simulink model "QRLsimbranch"  (R2013b)
settings: Solver=ode3  StartTime=0.0  StopTime=Tsim_end  FixedStep=Tsim_s  RelTol=1e-3
values from neighbouring files (symbols this model uses):
  b = 0.1    [QRLrunfile.m]    (also in hat.m = vec(2))
  b1d = [1; 0; 0]    [QRLrunfile.m]
  ctauf = 8.004e-3    (= 0.008004)    [QRLrunfile.m]
  d = 0.1    [QRLrunfile.m]
  dq0 = [0;0;0]    [QRLrunfile.m]
  dxL0 = 0    [QRLrunfile.m]
  dyL0 = 0    [QRLrunfile.m]
  dzL0 = 0    [QRLrunfile.m]
  e3 = [0;0;1]    [QRLrunfile.m]
  fsat = 4*1.96*[1 -1]    [QRLrunfile.m]
  g = 9.81    [LQRrunfile.m]    (also in QRLrunfile.m)
  I = diag([Ixx Iyy Izz])    [QRLrunfile.m]
  Ir = 0.5    [QRLrunfile.m]
  Ixx = 0.0820    (= 0.082)    [LQRrunfile.m]    (also in QRLrunfile.m = 0.00223)
  Iyy = 0.0845    [LQRrunfile.m]    (also in QRLrunfile.m = 0.00299)
  Izz = 0.1377    [LQRrunfile.m]    (also in QRLrunfile.m = 0.0048)
  K = lqr(LQRA,LQRB,LQRQ,LQRR)    [LQRrunfile.m]
  kdx = 2.75    [QRLrunfile.m]
  komega = 0.1    [QRLQRATT-18-Apr-2017.mat]    (also in QRLrunfile.m = 2; savename.mat)
  kOmega = 0.1    [QRLrunfile.m]
  kpx = 6    [QRLrunfile.m]
  kq = 4    [QRLQRATT-18-Apr-2017.mat]    (also in QRLrunfile.m = 3.9; savename.mat)
  kR = 8.81    [QRLQRATT-18-Apr-2017.mat]    (also in QRLrunfile.m = 0.9; savename.mat)
  L = 0.7    [QRLrunfile.m]
  l = 0.126    [QRLrunfile.m]
  LQRA = [zeros(8) eye(8) ... (first row only)    [LQRrunfile.m]
  LQRB = [zeros(10,4) ... (first row only)    [LQRrunfile.m]
  LQRC = eye(16)    [LQRrunfile.m]
  mL = 0.1    [LQRrunfile.m]    (also in QRLrunfile.m)
  mode = 4    [QRLrunfile.m]
  mQ = 4.34    [LQRrunfile.m]    (also in QRLrunfile.m = 0.4)
  Msat = 2*l*1.96*[1 -1]    [QRLrunfile.m]
  phiL0 = deg2rad(0)    [QRLrunfile.m]
  pQ0 = 0    [QRLrunfile.m]
  psiL0 = 0    [QRLrunfile.m]
  q0 = [0 0 -1]    [QRLQRATT-18-Apr-2017.mat]    (also in QRLrunfile.m = Rzyx*e3*qmode; savename.mat)
  qd = [0; 0; qmode]    [QRLrunfile.m]
  qmode = -1    [QRLrunfile.m]
  qQ0 = 0    [QRLrunfile.m]
  R0 = [1  0  0; 0  0.5  -0.866025403784; 0  0.866025403784  0.5]    [QRLQRATT-18-Apr-2017.mat]    (also in QRLrunfile.m = Rzyx; savename.mat)
  Rd = eye(3)    [QRLrunfile.m]
  rQ0 = 0    [QRLrunfile.m]
  stepamp = 0.25    [QRLrunfile.m]
  stept = 1    [QRLrunfile.m]
  thetaL0 = deg2rad(0)    [QRLrunfile.m]
  xL0 = q0(1)*L    [QRLrunfile.m]
  yL0 = q0(2)*L    [QRLrunfile.m]
  zL0 = L+q0(3)*L    [QRLrunfile.m]
undefined symbols (not defined in the file or in its folder): lqr0, sigbuilder_block, T0
libraries: simulink_extras x8, CF3 x7, vrlib x5, simulink x5, dspmathops x3, aerolibtransform2 x2, CommandFilter x1
(part 2 of 2)

== system QRLsimbranch/Trajectory/Path/Sines/Sine diagonal ==
  Add : Sum
  Add1 : Sum
  Add2 : Sum
  Gain : Gain
  Gain1 : Gain
  Gain2 : Gain
  Mux1 : Mux  Inputs=3
  Product : Product
  Product2 : Product
  Product6 : Product
  Scope3 : Scope  NumInputPorts=3
      settings: YMin=-5~-5~-5  YMax=5~5~5  SaveName=ScopeData24
  Signal Builder : Subsystem  Tag=STV Subsys  LoadFcn=sigbuilder_block('load');  StartFcn=sigbuilder_block('start');  StopFcn=sigbuilder_block('stop');  ClipboardFcn=sigbuilder_block('clipboard');  mask(Sigbuilder block){}
      mask help: Simulink:masks:SigbuilderBlock_MD
      mask init:
      | if ~strcmp(get_param(bdroot(gcbh),'SimulationStatus'),'stopped') tuvar = sigbuilder_block('maskInit'); end
      settings: CopyFcn=sigbuilder_block('copy');  DeleteFcn=sigbuilder_block('delete');  ModelCloseFcn=sigbuilder_block('modelClose');  PreSaveFcn=sigbuilder_block('preSave');  PauseFcn=sigbuilder_block('pause');  ContinueFcn=sigbuilder_block('continue');  NameChangeFcn=sigbuilder_block('namechange');  OpenFcn=sigbuilder_block('open',[0 222 1024.5 489 ]);  CloseFcn=sigbuilder_block('close');
      mask Display: plot(0, 0, 100, 100,[2, 2, 32, 32, 2], [68, 8, 8, 68, 68],[32, 2], [38, 38], [32, 19, 2],[53, 60, 44], [32, 17, 17, 2],[16, 16, 31, 31]);txt = getActiveGroup(gcbh);text(2, 100, txt,'verticalAlignment', 'top');
  Sine Wave7 : Sin  Bias=1  Frequency=2*pi/20  Phase=pi  SampleTime=0
  Sine Wave8 : Sin  Amplitude=0.25  Bias=0.25  Frequency=2*pi/3  SampleTime=0
  Sine Wave9 : Sin  Amplitude=0.25  Bias=0.25  Frequency=2*pi/3  SampleTime=0
  Out1 : Outport
  wires:
  Sine Wave7/1 -> Product/1, Scope3/1
  Add2/1 -> Gain/1
  Mux1/1 -> Out1/1
  Signal Builder/3(Signal 3) -> Product2/2
  Signal Builder/2(Signal 2) -> Add/2
  Product6/1 -> Add2/1
  Add/1 -> Gain2/1
  Signal Builder/1(Signal 1) -> Product/2
  Product/1 -> Add/1
  Gain/1 -> Mux1/3
  Sine Wave9/1 -> Scope3/3, Product6/1
  Add1/1 -> Gain1/1
  Gain1/1 -> Mux1/2
  Signal Builder/5(Signal 5) -> Product6/2
  Product2/1 -> Add1/1
  Sine Wave8/1 -> Product2/1, Scope3/2
  Gain2/1 -> Mux1/1

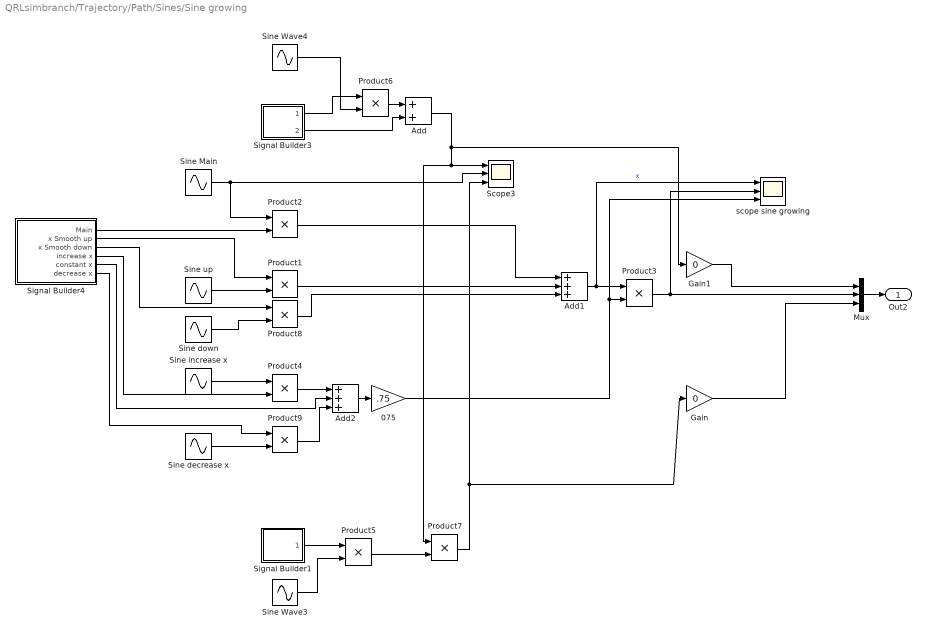
== system QRLsimbranch/Trajectory/Path/Sines/Sine growing ==
  075 : Gain  Gain=.75
  Add : Sum
  Add1 : Sum  Inputs=+++
  Add2 : Sum  Inputs=+++
  Gain : Gain  Gain=0
  Gain1 : Gain  Gain=0
  Mux : Mux  Inputs=3
  Product{1..9} (9 alike) : Product
  Scope3 : Scope  NumInputPorts=3
      settings: YMin=0~-1~0  YMax=0.9~1~0.45  SaveName=ScopeData54
  Signal Builder1 : Subsystem  Tag=STV Subsys  LoadFcn=sigbuilder_block('load');  StartFcn=sigbuilder_block('start');  StopFcn=sigbuilder_block('stop');  ClipboardFcn=sigbuilder_block('clipboard');  mask(Sigbuilder block){}
      mask help: Simulink:masks:SigbuilderBlock_MD
      mask init:
      | if ~strcmp(get_param(bdroot(gcbh),'SimulationStatus'),'stopped') tuvar = sigbuilder_block('maskInit'); end
      settings: CopyFcn=sigbuilder_block('copy');  DeleteFcn=sigbuilder_block('delete');  ModelCloseFcn=sigbuilder_block('modelClose');  PreSaveFcn=sigbuilder_block('preSave');  PauseFcn=sigbuilder_block('pause');  ContinueFcn=sigbuilder_block('continue');  NameChangeFcn=sigbuilder_block('namechange');  OpenFcn=sigbuilder_block('open',[6 28.5 1012.5 484.5 ]);  CloseFcn=sigbuilder_block('close');
      mask Display: plot(0, 0, 100, 100,[2, 2, 32, 32, 2], [68, 8, 8, 68, 68],[32, 2], [38, 38], [32, 19, 2],[53, 60, 44], [32, 17, 17, 2],[16, 16, 31, 31]);txt = getActiveGroup(gcbh);text(2, 100, txt,'verticalAlignment', 'top');
  Signal Builder3 : Subsystem  Tag=STV Subsys  LoadFcn=sigbuilder_block('load');  StartFcn=sigbuilder_block('start');  StopFcn=sigbuilder_block('stop');  ClipboardFcn=sigbuilder_block('clipboard');  mask(Sigbuilder block){}
      mask help: Simulink:masks:SigbuilderBlock_MD
      mask init:
      | if ~strcmp(get_param(bdroot(gcbh),'SimulationStatus'),'stopped') tuvar = sigbuilder_block('maskInit'); end
      settings: CopyFcn=sigbuilder_block('copy');  DeleteFcn=sigbuilder_block('delete');  ModelCloseFcn=sigbuilder_block('modelClose');  PreSaveFcn=sigbuilder_block('preSave');  PauseFcn=sigbuilder_block('pause');  ContinueFcn=sigbuilder_block('continue');  NameChangeFcn=sigbuilder_block('namechange');  OpenFcn=sigbuilder_block('open',[6 28.5 1012.5 484.5 ]);  CloseFcn=sigbuilder_block('close');
      mask Display: plot(0, 0, 100, 100,[2, 2, 32, 32, 2], [68, 8, 8, 68, 68],[32, 2], [38, 38], [32, 19, 2],[53, 60, 44], [32, 17, 17, 2],[16, 16, 31, 31]);txt = getActiveGroup(gcbh);text(2, 100, txt,'verticalAlignment', 'top');
  Signal Builder4 : Subsystem  Tag=STV Subsys  LoadFcn=sigbuilder_block('load');  StartFcn=sigbuilder_block('start');  StopFcn=sigbuilder_block('stop');  ClipboardFcn=sigbuilder_block('clipboard');  mask(Sigbuilder block){}
      mask help: Simulink:masks:SigbuilderBlock_MD
      mask init:
      | if ~strcmp(get_param(bdroot(gcbh),'SimulationStatus'),'stopped') tuvar = sigbuilder_block('maskInit'); end
      settings: CopyFcn=sigbuilder_block('copy');  DeleteFcn=sigbuilder_block('delete');  ModelCloseFcn=sigbuilder_block('modelClose');  PreSaveFcn=sigbuilder_block('preSave');  PauseFcn=sigbuilder_block('pause');  ContinueFcn=sigbuilder_block('continue');  NameChangeFcn=sigbuilder_block('namechange');  OpenFcn=sigbuilder_block('open',[518.25 228 500.25 477 ]);  CloseFcn=sigbuilder_block('close');
      mask Display: plot(0, 0, 100, 100,[2, 2, 32, 32, 2], [68, 8, 8, 68, 68],[32, 2], [38, 38], [32, 19, 2],[53, 60, 44], [32, 17, 17, 2],[16, 16, 31, 31]);txt = getActiveGroup(gcbh);text(2, 100, txt,'verticalAlignment', 'top');
  Sine Main : Sin  Frequency=2*pi/3  SampleTime=0
  Sine Wave3 : Sin  Amplitude=0.5/2  Bias=0.5/2  Frequency=2*pi/1.5  Phase=1.5*pi  SampleTime=0
  Sine Wave4 : Sin  Amplitude=0.5  Bias=0.5  Frequency=2*pi/40  Phase=1.5*pi  SampleTime=0
  Sine decrease x : Sin  Amplitude=.5  Bias=.5  Frequency=2*pi/20  Phase=1*pi  SampleTime=0
  Sine down : Sin  Amplitude=.5  Bias=.5  Frequency=2*pi/3  Phase=0*pi  SampleTime=0
  Sine increase x : Sin  Amplitude=.5  Bias=.5  Frequency=2*pi/20  Phase=1.5*pi  SampleTime=0
  Sine up : Sin  Amplitude=.5  Bias=.5  Frequency=2*pi/1.5  Phase=1.5*pi  SampleTime=0
  scope sine growing : Scope  NumInputPorts=3
      settings: YMin=-5~-5~-5  YMax=5~5~5  SaveName=ScopeData55
  Out2 : Outport
  wires:
  Add1/1 -> scope sine growing/1, Product3/1  "x"
  Product2/1 -> Add1/1
  Sine Main/1 -> Scope3/2, Product2/1
  Product1/1 -> Add1/2
  Product3/1 -> scope sine growing/2, Mux/2
  Mux/1 -> Out2/1
  Add2/1 -> 075/1
  Signal Builder1/1(Signal 3) -> Product5/1
  Sine Wave3/1 -> Product5/2
  Signal Builder3/1(Signal 3) -> Product6/1
  Sine Wave4/1 -> Product6/2
  Product6/1 -> Add/1
  Signal Builder3/2(Signal 1) -> Add/2
  Add/1 -> Product7/1, Scope3/1, Gain1/1
  Gain1/1 -> Mux/1
  Product7/1 -> Scope3/3, Gain/1
  Gain/1 -> Mux/3
  Product5/1 -> Product7/2
  Signal Builder4/1(Main) -> Product2/2
  Signal Builder4/2(x Smooth up) -> Product1/1
  Sine up/1 -> Product1/2
  Product8/1 -> Add1/3
  Signal Builder4/3(x Smooth down) -> Product8/1
  Sine down/1 -> Product8/2
  Product4/1 -> Add2/1
  Sine increase x/1 -> Product4/1
  Signal Builder4/4(increase x) -> Product4/2
  Sine decrease x/1 -> Product9/2
  075/1 -> scope sine growing/3, Product3/2
  Signal Builder4/6(decrease x) -> Product9/1
  Signal Builder4/5(constant x) -> Add2/2
  Product9/1 -> Add2/3

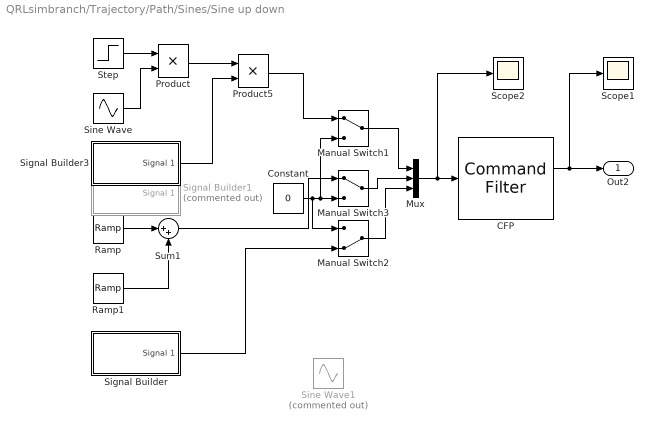
== system QRLsimbranch/Trajectory/Path/Sines/Sine up down ==
  CFP : CF3/Command Filter  Integrator1_init=0  omega_n1=omega_n1_CFP  omega_n2=omega_n2_CFP  zeta=zeta_xL
  Constant : Constant  Value=0
  Manual Switch1 : ManualSwitch
  Manual Switch2 : ManualSwitch  CurrentSetting=0
  Manual Switch3 : ManualSwitch
  Mux : Mux  Inputs=3
  Product : Product
  Product5 : Product
  Ramp : simulink/Sources/Ramp  slope=1/2  start=0  X0=0
  Ramp1 : simulink/Sources/Ramp  slope=-1/2  start=14  X0=0
  Scope1 : Scope
      settings: SaveName=ScopeData8
  Scope2 : Scope
      settings: SaveName=ScopeData50
  Signal Builder : Subsystem  Tag=STV Subsys  LoadFcn=sigbuilder_block('load');  StartFcn=sigbuilder_block('start');  StopFcn=sigbuilder_block('stop');  ClipboardFcn=sigbuilder_block('clipboard');  mask(Sigbuilder block){}
      mask help: Simulink:masks:SigbuilderBlock_MD
      mask init:
      | if ~strcmp(get_param(bdroot(gcbh),'SimulationStatus'),'stopped') tuvar = sigbuilder_block('maskInit'); end
      settings: CopyFcn=sigbuilder_block('copy');  DeleteFcn=sigbuilder_block('delete');  ModelCloseFcn=sigbuilder_block('modelClose');  PreSaveFcn=sigbuilder_block('preSave');  PauseFcn=sigbuilder_block('pause');  ContinueFcn=sigbuilder_block('continue');  NameChangeFcn=sigbuilder_block('namechange');  OpenFcn=sigbuilder_block('open',[611.25 186.75 750 399.75 ]);  CloseFcn=sigbuilder_block('close');
      mask Display: plot(0, 0, 100, 100,[2, 2, 32, 32, 2], [68, 8, 8, 68, 68],[32, 2], [38, 38], [32, 19, 2],[53, 60, 44], [32, 17, 17, 2],[16, 16, 31, 31]);txt = getActiveGroup(gcbh);text(2, 100, txt,'verticalAlignment', 'top');
  Signal Builder1 : Subsystem  Tag=STV Subsys  Commented=on  LoadFcn=sigbuilder_block('load');  StartFcn=sigbuilder_block('start');  StopFcn=sigbuilder_block('stop');  ClipboardFcn=sigbuilder_block('clipboard');  mask(Sigbuilder block){}
      mask help: Simulink:masks:SigbuilderBlock_MD
      mask init:
      | if ~strcmp(get_param(bdroot(gcbh),'SimulationStatus'),'stopped') tuvar = sigbuilder_block('maskInit'); end
      settings: CopyFcn=sigbuilder_block('copy');  DeleteFcn=sigbuilder_block('delete');  ModelCloseFcn=sigbuilder_block('modelClose');  PreSaveFcn=sigbuilder_block('preSave');  PauseFcn=sigbuilder_block('pause');  ContinueFcn=sigbuilder_block('continue');  NameChangeFcn=sigbuilder_block('namechange');  OpenFcn=sigbuilder_block('open',[6 213.75 948 395.25 ]);  CloseFcn=sigbuilder_block('close');
      mask Display: plot(0, 0, 100, 100,[2, 2, 32, 32, 2], [68, 8, 8, 68, 68],[32, 2], [38, 38], [32, 19, 2],[53, 60, 44], [32, 17, 17, 2],[16, 16, 31, 31]);txt = getActiveGroup(gcbh);text(2, 100, txt,'verticalAlignment', 'top');
  Signal Builder3 : Subsystem  Tag=STV Subsys  LoadFcn=sigbuilder_block('load');  StartFcn=sigbuilder_block('start');  StopFcn=sigbuilder_block('stop');  ClipboardFcn=sigbuilder_block('clipboard');  mask(Sigbuilder block){}
      mask help: Simulink:masks:SigbuilderBlock_MD
      mask init:
      | if ~strcmp(get_param(bdroot(gcbh),'SimulationStatus'),'stopped') tuvar = sigbuilder_block('maskInit'); end
      settings: CopyFcn=sigbuilder_block('copy');  DeleteFcn=sigbuilder_block('delete');  ModelCloseFcn=sigbuilder_block('modelClose');  PreSaveFcn=sigbuilder_block('preSave');  PauseFcn=sigbuilder_block('pause');  ContinueFcn=sigbuilder_block('continue');  NameChangeFcn=sigbuilder_block('namechange');  OpenFcn=sigbuilder_block('open',[6 213.75 948 395.25 ]);  CloseFcn=sigbuilder_block('close');
      mask Display: plot(0, 0, 100, 100,[2, 2, 32, 32, 2], [68, 8, 8, 68, 68],[32, 2], [38, 38], [32, 19, 2],[53, 60, 44], [32, 17, 17, 2],[16, 16, 31, 31]);txt = getActiveGroup(gcbh);text(2, 100, txt,'verticalAlignment', 'top');
  Sine Wave : Sin  Frequency=2*pi/2.5  SampleTime=0
  Sine Wave1 : Sin  Commented=on  Frequency=2*pi/2.5*2  Phase=pi  SampleTime=0
  Step : Step  Time=0  After=.5  SampleTime=0
  Sum1 : Sum  Inputs=|++
  Out2 : Outport
  wires:
  Mux/1 -> Scope2/1, CFP/1
  Constant/1 -> Manual Switch3/2, Manual Switch1/2, Manual Switch2/1
  Manual Switch1/1 -> Mux/1
  Manual Switch2/1 -> Mux/3
  Ramp/1 -> Sum1/1
  Manual Switch3/1 -> Mux/2
  Step/1 -> Product/1
  Sine Wave/1 -> Product/2
  Product/1 -> Product5/1
  Product5/1 -> Manual Switch1/1
  Ramp1/1 -> Sum1/2
  Sum1/1 -> Manual Switch3/1
  CFP/2 -> Scope1/1, Out2/1
  Signal Builder/1(Signal 1) -> Manual Switch2/2
  Signal Builder3/1(Signal 1) -> Product5/2

== system QRLsimbranch/Trajectory/Path/Square/Signal Builder3 ==
  Demux : Demux  Tag=STV Demux  Outputs=2
  FromWs : FromWorkspace  Tag=STV FromWs  VariableName=tuvar  SampleTime=0
      SigBuilderData=|
      | common.afterFinalStr = 'Extrapolate'
      | common.sampleTime = 0
      | dataSet.timeRange = [0 20]
      | dataSet.name = 'Group 1'
      | sbobj.Groups.Name = 'Group 1'
      | sbobj.Groups.Signals(1).Name = 'Signal 1'
      | sbobj.Groups.Signals(1).XData = [0 1 5 9 13 20]
      | sbobj.Groups.Signals(1).YData = [0 0 1 1 0 0]
      | sbobj.Groups.Signals(2).Name = 'Signal 2'
      | sbobj.Groups.Signals(2).XData = [0 5 9 13 17 20]
      | sbobj.Groups.Signals(2).YData = [0 0 1 1 0 0]
      | sbobj.Groups.TimeRange = [0 20]
  Signal 1 : Outport  Tag=STV Outport
  Signal 2 : Outport  Tag=STV Outport  Port=2
  wires:
  Demux/1 -> Signal 1/1
  FromWs/1 -> Demux/1
  Demux/2 -> Signal 2/1

== system QRLsimbranch/Trajectory/Step/step3dir/Signal Builder ==
  Demux : Demux  Tag=STV Demux  Outputs=6
  FromWs : FromWorkspace  Tag=STV FromWs  VariableName=tuvar  SampleTime=0
      SigBuilderData=|
      | common.afterFinalStr = 'Extrapolate'
      | common.sampleTime = 0
      | dataSet.timeRange = [0 15]
      | dataSet.name = 'Group 1'
      | sbobj.Groups.Name = 'Group 1'
      | sbobj.Groups.Signals(1).Name = 'Signal 1'
      | sbobj.Groups.Signals(1).XData = [0 1 1 4 4 15]
      | sbobj.Groups.Signals(1).YData = [0 0 1 1 0 0]
      | sbobj.Groups.Signals(2).Name = 'Signal 2'
      | sbobj.Groups.Signals(2).XData = [0 4 4 15]
      | sbobj.Groups.Signals(2).YData = [0 0 1 1]
      | sbobj.Groups.Signals(3).Name = 'Signal 3'
      | sbobj.Groups.Signals(3).XData = [0 4.5 4.5 7.5 7.5 15]
      | sbobj.Groups.Signals(3).YData = [0 0 1 1 0 0]
      | sbobj.Groups.Signals(4).Name = 'Signal 4'
      | sbobj.Groups.Signals(4).XData = [0 7.5 7.5 15]
      | sbobj.Groups.Signals(4).YData = [0 0 1 1]
      | sbobj.Groups.Signals(5).Name = 'Signal 5'
      | sbobj.Groups.Signals(5).XData = [0 8 8 11 11 15]
      | sbobj.Groups.Signals(5).YData = [0 0 1 1 0 0]
      | sbobj.Groups.Signals(6).Name = 'Signal 6'
      | sbobj.Groups.Signals(6).XData = [0 11 11 15]
      | sbobj.Groups.Signals(6).YData = [0 0 1 1]
      | sbobj.Groups.TimeRange = [0 15]
  Signal 1 : Outport  Tag=STV Outport
  Signal 2 : Outport  Tag=STV Outport  Port=2
  Signal 3 : Outport  Tag=STV Outport  Port=3
  Signal 4 : Outport  Tag=STV Outport  Port=4
  Signal 5 : Outport  Tag=STV Outport  Port=5
  Signal 6 : Outport  Tag=STV Outport  Port=6
  wires:
  Demux/1 -> Signal 1/1
  FromWs/1 -> Demux/1
  Demux/2 -> Signal 2/1
  Demux/3 -> Signal 3/1
  Demux/4 -> Signal 4/1
  Demux/5 -> Signal 5/1
  Demux/6 -> Signal 6/1

== system QRLsimbranch/Trajectory/Path/Sines/Sine diagonal/Signal Builder ==
  Demux : Demux  Tag=STV Demux  Outputs=6
  FromWs : FromWorkspace  Tag=STV FromWs  VariableName=tuvar  SampleTime=0
      SigBuilderData=|
      | common.afterFinalStr = 'Extrapolate'
      | common.sampleTime = 0
      | dataSet.timeRange = [0 21]
      | dataSet.name = 'Group 1'
      | sbobj.Groups.Name = 'Group 1'
      | sbobj.Groups.Signals(1).Name = 'Signal 1'
      | sbobj.Groups.Signals(1).XData = [0 5 5 15 15 21]
      | sbobj.Groups.Signals(1).YData = [0 0 1 1 0 0]
      | sbobj.Groups.Signals(2).Name = 'Signal 2'
      | sbobj.Groups.Signals(2).XData = [0 15 15 21]
      | sbobj.Groups.Signals(2).YData = [0 0 2 2]
      | sbobj.Groups.Signals(3).Name = 'Signal 3'
      | sbobj.Groups.Signals(3).XData = [0 5.25 5.25 14.25 14.25 21]
      | sbobj.Groups.Signals(3).YData = [0 0 1 1 0 0]
      | sbobj.Groups.Signals(4).Name = 'Signal 4'
      | sbobj.Groups.Signals(4).XData = [0 7.5 21]
      | sbobj.Groups.Signals(4).YData = [0 0 0]
      | sbobj.Groups.Signals(5).Name = 'Signal 5'
      | sbobj.Groups.Signals(5).XData = [0 5.25 5.25 14.25 14.25 21]
      | sbobj.Groups.Signals(5).YData = [0 0 1 1 0 0]
      | sbobj.Groups.Signals(6).Name = 'Signal 6'
      | sbobj.Groups.Signals(6).XData = [0 11 21]
      | sbobj.Groups.Signals(6).YData = [0 0 0]
      | sbobj.Groups.TimeRange = [0 21]
  Signal 1 : Outport  Tag=STV Outport
  Signal 2 : Outport  Tag=STV Outport  Port=2
  Signal 3 : Outport  Tag=STV Outport  Port=3
  Signal 4 : Outport  Tag=STV Outport  Port=4
  Signal 5 : Outport  Tag=STV Outport  Port=5
  Signal 6 : Outport  Tag=STV Outport  Port=6
  wires:
  Demux/1 -> Signal 1/1
  FromWs/1 -> Demux/1
  Demux/2 -> Signal 2/1
  Demux/3 -> Signal 3/1
  Demux/4 -> Signal 4/1
  Demux/5 -> Signal 5/1
  Demux/6 -> Signal 6/1

== system QRLsimbranch/Trajectory/Path/Sines/Sine growing/Signal Builder1 ==
  Demux : Demux  Tag=STV Demux  Outputs=1
  FromWs : FromWorkspace  Tag=STV FromWs  VariableName=tuvar  SampleTime=0
      SigBuilderData=|
      | common.afterFinalStr = 'Extrapolate'
      | common.sampleTime = 0
      | dataSet.timeRange = [0 21]
      | dataSet.name = 'Group 1'
      | sbobj.Groups.Name = 'Group 1'
      | sbobj.Groups.Signals.Name = 'Signal 3'
      | sbobj.Groups.Signals.XData = [0 3 3 20 20 21]
      | sbobj.Groups.Signals.YData = [0 0 0.65 0.65 0 0]
      | sbobj.Groups.TimeRange = [0 21]
  Signal 3 : Outport  Tag=STV Outport
  wires:
  FromWs/1 -> Demux/1
  Demux/1 -> Signal 3/1

== system QRLsimbranch/Trajectory/Path/Sines/Sine growing/Signal Builder3 ==
  Demux : Demux  Tag=STV Demux  Outputs=2
  FromWs : FromWorkspace  Tag=STV FromWs  VariableName=tuvar  SampleTime=0
      SigBuilderData=|
      | common.afterFinalStr = 'Extrapolate'
      | common.sampleTime = 0
      | dataSet.timeRange = [0 21]
      | dataSet.name = 'Group 1'
      | sbobj.Groups.Name = 'Group 1'
      | sbobj.Groups.Signals(1).Name = 'Signal 3'
      | sbobj.Groups.Signals(1).XData = [0 20 20 21]
      | sbobj.Groups.Signals(1).YData = [1 1 0 0]
      | sbobj.Groups.Signals(2).Name = 'Signal 1'
      | sbobj.Groups.Signals(2).XData = [0 20 20 21]
      | sbobj.Groups.Signals(2).YData = [0 0 1 1]
      | sbobj.Groups.TimeRange = [0 21]
  Signal 3 : Outport  Tag=STV Outport
  Signal 1 : Outport  Tag=STV Outport  Port=2
  wires:
  FromWs/1 -> Demux/1
  Demux/1 -> Signal 3/1
  Demux/2 -> Signal 1/1

== system QRLsimbranch/Trajectory/Path/Sines/Sine growing/Signal Builder4 ==
  Demux : Demux  Tag=STV Demux  Outputs=6
  FromWs : FromWorkspace  Tag=STV FromWs  VariableName=tuvar  SampleTime=0
      SigBuilderData=|
      | common.afterFinalStr = 'Extrapolate'
      | common.sampleTime = 0
      | dataSet.timeRange = [0 25]
      | dataSet.name = 'Group 1'
      | sbobj.Groups.Name = 'Group 1'
      | sbobj.Groups.Signals(1).Name = 'Main'
      | sbobj.Groups.Signals(1).XData = [0 0.75 0.75 21.75 21.75 25]
      | sbobj.Groups.Signals(1).YData = [0 0 1 1 0 0]
      | sbobj.Groups.Signals(2).Name = 'x Smooth up'
      | sbobj.Groups.Signals(2).XData = [0 0.75 0.75 25]
      | sbobj.Groups.Signals(2).YData = [1 1 0 0]
      | sbobj.Groups.Signals(3).Name = 'x Smooth down'
      | sbobj.Groups.Signals(3).XData = [0 21.75 21.75 23.25 23.25 25]
      | sbobj.Groups.Signals(3).YData = [0 0 1 1 0 0]
      | sbobj.Groups.Signals(4).Name = 'increase x'
      | sbobj.Groups.Signals(4).XData = [0 10 10 25]
      | sbobj.Groups.Signals(4).YData = [1 1 0 0]
      | sbobj.Groups.Signals(5).Name = 'constant x'
      | sbobj.Groups.Signals(5).XData = [0 10 10 15 15 25]
      | sbobj.Groups.Signals(5).YData = [0 0 1 1 0 0]
      | sbobj.Groups.Signals(6).Name = 'decrease x'
      | sbobj.Groups.Signals(6).XData = [0 15 15 25]
      | sbobj.Groups.Signals(6).YData = [0 0 1 1]
      | sbobj.Groups.TimeRange = [0 25]
  Main : Outport  Tag=STV Outport
  x Smooth up : Outport  Tag=STV Outport  Port=2
  x Smooth down : Outport  Tag=STV Outport  Port=3
  increase x : Outport  Tag=STV Outport  Port=4
  constant x : Outport  Tag=STV Outport  Port=5
  decrease x : Outport  Tag=STV Outport  Port=6
  wires:
  FromWs/1 -> Demux/1
  Demux/1 -> Main/1
  Demux/2 -> x Smooth up/1
  Demux/3 -> x Smooth down/1
  Demux/4 -> increase x/1
  Demux/5 -> constant x/1
  Demux/6 -> decrease x/1

== system QRLsimbranch/Trajectory/Path/Sines/Sine up down/Signal Builder ==
  Demux : Demux  Tag=STV Demux  Outputs=1
  FromWs : FromWorkspace  Tag=STV FromWs  VariableName=tuvar  SampleTime=0
      SigBuilderData=|
      | common.afterFinalStr = 'Extrapolate'
      | common.sampleTime = 0
      | dataSet.timeRange = [0 15]
      | dataSet.name = 'Group 1'
      | sbobj.Groups.Name = 'Group 1'
      | sbobj.Groups.Signals.Name = 'Signal 1'
      | sbobj.Groups.Signals.XData = [0 2 7.5 12.5 15]
      | sbobj.Groups.Signals.YData = [0 0 1 0 0]
      | sbobj.Groups.TimeRange = [0 15]
  Signal 1 : Outport  Tag=STV Outport
  wires:
  Demux/1 -> Signal 1/1
  FromWs/1 -> Demux/1

== system QRLsimbranch/Trajectory/Path/Sines/Sine up down/Signal Builder1 ==
  Demux : Demux  Tag=STV Demux  Outputs=1
  FromWs : FromWorkspace  Tag=STV FromWs  VariableName=tuvar  SampleTime=0
      SigBuilderData=|
      | common.afterFinalStr = 'Extrapolate'
      | common.sampleTime = 0
      | dataSet.timeRange = [0 20]
      | dataSet.name = 'Group 1'
      | sbobj.Groups.Name = 'Group 1'
      | sbobj.Groups.Signals.Name = 'Signal 1'
      | sbobj.Groups.Signals.XData = [0 20]
      | sbobj.Groups.Signals.YData = [1 1]
      | sbobj.Groups.TimeRange = [0 20]
  Signal 1 : Outport  Tag=STV Outport
  wires:
  Demux/1 -> Signal 1/1
  FromWs/1 -> Demux/1

== system QRLsimbranch/Trajectory/Path/Sines/Sine up down/Signal Builder3 ==
  Demux : Demux  Tag=STV Demux  Outputs=1
  FromWs : FromWorkspace  Tag=STV FromWs  VariableName=tuvar  SampleTime=0
      SigBuilderData=|
      | common.afterFinalStr = 'Extrapolate'
      | common.sampleTime = 0
      | dataSet.timeRange = [0 20]
      | dataSet.name = 'Group 1'
      | sbobj.Groups.Name = 'Group 1'
      | sbobj.Groups.Signals.Name = 'Signal 1'
      | sbobj.Groups.Signals.XData = [0 1 5 9 13 20]
      | sbobj.Groups.Signals.YData = [0 0 1.25 1.25 0 0]
      | sbobj.Groups.TimeRange = [0 20]
  Signal 1 : Outport  Tag=STV Outport
  wires:
  Demux/1 -> Signal 1/1
  FromWs/1 -> Demux/1

== matlab function QRLsimbranch/QR-Load Nonlinear model/q block1/MATLAB Function1 ==
  data: q input; normq output
function normq = fcn(q)
%#codegen

normq = norm(q);

== matlab function QRLsimbranch/QR-Load Nonlinear model/q block1/MATLAB Function2 ==
  data: R input; detR output
function detR = fcn(R)
%#codegen

detR = det(R);

== matlab function QRLsimbranch/Control Nonlinear Geometric/QRL Load Attitude Controller/Subsystem/MATLAB Function ==
  data: C input; dRc output; dC input; ddC input; b3c input; F input; dF input; ddF input; ddRc output
function [dRc,ddRc] = fcn(C,dC,ddC,b3c,F,dF,ddF)
%#codegen

b2c = C/norm(C);

db3c = dF/norm(F) + dot(F,dF)*F/norm(F)^3;
db2c = dC/norm(C) + dot(C,dC)*C/norm(C)^3;
db1c = cross(db2c,b3c) + cross(b2c,db3c);
dRc = [db1c db2c db3c];

ddb3c = ddF/norm(F) + 2*dot(F,dF)*dF/norm(F)^3 + (norm(dF)^2+dot(F,ddF))*F/norm(F)^3 - 3*dot(F,dF)^2*F/norm(F)^5;
ddb2c = ddC/norm(C) + 2*dot(C,dC)*dC/norm(C)^3 + (norm(dC)^2+dot(C,ddC))*C/norm(C)^3 - 3*dot(C,dC)^2*C/norm(C)^5;
ddb1c = cross(ddb2c,b3c) + 2*cross(db2c,db3c) + cross(b2c,ddb3c);
ddRc = [ddb1c ddb2c ddb3c];

== matlab function QRLsimbranch/QR-Load Nonlinear model/Integration Block/MATLAB Function ==
  data: q input; anglesL output
function anglesL = fcn(q)
%#codegen
x = q(1);
y = q(2);
z = q(3);

% phiL = acos(-z);
% thetaL = atan2(y,x);
phiL = asin(y);
thetaL = asin(x);
psiL = 0;

anglesL = [phiL;thetaL;psiL];

== matlab function QRLsimbranch/Control LQR/MATLAB Function ==
  data: u input; xL output; xQ input
function xL = fcn(u,xQ)
%#codegen

theL = u(2);
phiL = u(1);

L = 0.7;

% x = L*sin(theL)*cos(phiL);
% y = L*sin(theL)*sin(phiL);
% z = -L*cos(theL);

x=L*sin(theL);
y=L*sin(phiL);
z=-L*cos(theL)*cos(phiL);

xL = xQ+[x;y;z];

== matlab function QRLsimbranch/QR-Load Nonlinear model/R block/dR block ==
  data: R input size=[3 3]; dR output size=[3 3]; Omega input size=3
function dR = fcn(R,Omega)
%#codegen
p = Omega(1);
q = Omega(2);
r = Omega(3);

Omegahat = [0 -r  q;
            r  0 -p;
           -q  p  0];

dR = R*Omegahat;
% R1 = R;

== matlab function QRLsimbranch/QR-Load Nonlinear model/omegarot block/fcnomega ==
  data: var input; M input size=3; f input; omegai output size=4; fi output
function [omegai,fi] = fcn(var,M,f)
%omega = [omega_1^2;omega_2^2;omega_3^2;omega_4^2]

b = var(1);
d = var(2);
l = var(3);

%check if Gamma is invertible?
Gamma = [b b b b;0 -l*b 0 l*b;l*b 0 -l*b 0;-d d -d d];

QRinput = [f;M];

omegai = Gamma\QRinput;
fi = b*omegai;

== matlab function QRLsimbranch/QR-Load Nonlinear model/dxL block ==
  data: varddxL input; q input size=3; dq input; ddxL output size=3; R input size=[3 3]; f input size=1
function ddxL = fcn(varddxL,q,dq,R,f)

mQ = varddxL(1);
g  = varddxL(2);
mL = varddxL(3);
L = varddxL(4);

e3 = [0;0;1];



ddxL = ( ( (dot(q,(f*R*e3)) - mQ*L*dot(dq,dq)) * q ) / (mQ+mL) ) - g*e3;

== matlab function QRLsimbranch/QR-Load Nonlinear model/q block1/MATLAB Function ==
  data: q input; OmegaL output; dq input
function OmegaL = fcn(q,dq)
%#codegen

qhat = [0 -q(3) q(2);
        q(3) 0 -q(1);
        -q(2) q(1) 0];


OmegaL = qhat*dq;

== matlab function QRLsimbranch/Control Nonlinear Geometric/QRL QR Attitude Controller/eRhat block ==
  data: Rc input size=[3 3]; R input size=[3 3]; eR output size=3; PsiR output
function [eR,PsiR] = fcneRc(Rc,R)

eRhat = (Rc.'*R-R.'*Rc);
eR = 0.5*[eRhat(6);-eRhat(3);eRhat(2)]; 
PsiR = 0.5*trace(eye(3) - Rc.'*R);
% test = Rc.'*R;
% 
% for k = 1:length(Rc.signals.values)
%     test(:,:,k) = Rc.signals.values(:,:,k).'*Rc.signals.values(:,:,k);
% end

% test = diag(Rc.'*R);

== matlab function QRLsimbranch/Control Nonlinear Geometric/QRL Load Attitude Controller/Rc block ==
  data: b1d input size=[3 1]; Rc output size=[3 3]; b2c output; b3c input size=[3 1]; C output
function [Rc,b2c,C] = fcnRc(b1d,b3c)
%
b1c = -cross(b3c,cross(b3c,b1d)) / norm(cross(b3c,b1d));
% b1c = -cross(b3c,normc(cross(b3c,b1d)));
b2c = cross(b3c,b1c);
C = cross(b3c,b1d);
Rc = [b1c b2c b3c];
% Rc = Rc.';

== matlab function QRLsimbranch/Control Nonlinear Geometric/QRL QR Attitude Controller/eOmega block ==
  data: R input size=[3 3]; Rc input size=[3 3]; eOmega output size=3; Omega input size=[3 1]; Omegac input size=[3 1]
function eOmega = fcneOmega(R,Rc,Omega,Omegac)
% Z-X-Y psi-phi-theta

eOmega = Omega - R.'*Rc*Omegac;

== matlab function QRLsimbranch/Control Nonlinear Geometric/QRL QR Attitude Controller/Mterm Omegac/Omegac block ==
  data: Rc input size=[3 3]; dRc input size=[3 3]; Omegac output size=3; ddRc input; dOmegac output
function [Omegac,dOmegac] = fcnOmegac(Rc,dRc,ddRc)

Omegachat  = Rc.'*dRc;
Omegac     = [Omegachat(6);-Omegachat(3);Omegachat(2)];

dOmegachat = -Omegachat*Omegachat+Rc.'*ddRc;
dOmegac    = [dOmegachat(6);-dOmegachat(3);dOmegachat(2)];

== matlab function QRLsimbranch/Control Nonlinear Geometric/QRL QR Attitude Controller/Mterm Omegac/Subsystem1/M term block ==
  data: R input size=[3 3]; Rc input size=[3 3]; Out output size=3; Omega input size=3; Omegac input size=3; dOmegac input
function Out  = fcnMterm(R,Rc,Omega,Omegac,dOmegac)
% Z-X-Y psi-phi-theta

p = Omega(1);
q = Omega(2);
r = Omega(3);

Omegahat = [0 -r  q;
            r  0 -p;
           -q  p  0];
       
Out = Omegahat*R.'*Rc*Omegac - R.'*Rc*dOmegac;

== matlab function QRLsimbranch/Control Nonlinear Geometric/QRL Load Attitude Controller/MATLAB Function ==
  data: varF input; A input size=3; mode input; q input size=3; Fn output size=3; dq input size=3; qc input; dqc input; ddqc input; Fpd output size=3; Fff output size=3; eq output size=3; edq output size=3
function [Fn,Fpd,Fff,eq,edq] = Ffcn(varF,A,mode,q,dq,qc,dqc,ddqc)
kq = varF(1);
komega = varF(2);
mQ = varF(3);
L = varF(4);

switch mode
    case 4
        Fn = dot(A,q)*q;
    otherwise
        Fn = -dot(qc,q)*q;
end

qhat = [ 0    -q(3) q(2);  
         q(3)  0   -q(1);  
        -q(2)  q(1) 0];

eq = qhat^2*qc;
edq = dq - cross((cross(qc,dqc)),q);

Fpd = -kq*eq - komega*edq;


inprod = dot(q,(cross(qc,dqc)));% strange inproduct

Fff = mQ*L*inprod*cross(q,dq) + mQ*L*cross(cross(qc,ddqc),q);
% Fff = 0;
% Fff = mQ*inprod*cross(q,dq) + mQ*cross((cross(qc,ddqc)),q);

== matlab function QRLsimbranch/Control Nonlinear Geometric/QRL Load Attitude Controller/MATLAB Function1 ==
  data: q input; Psiq output; qc input
function Psiq = fcn(q,qc)

Psiq = 1 - qc'*q;
